simulink model "mavsim_chap3"  (R2021b)
settings: Solver=ode45  StartTime=0.0  StopTime=10000  RelTol=1e-3  EnableMultiTasking=on
InitFcn:
  | addpath('../chap2')
  | addpath('../parameters/')
  | aerosonde_parameters
undefined symbols (not defined in the file or in its folder): drawQuadrotor, plotmavstatevariables
libraries: simulink x7
settings Model: Creator=beard  LastModifiedBy=andrey
settings SolverCC: AlgebraicLoopSolver=TrustRegion
settings DataIOCC: LimitDataPoints=on  SaveFormat=Array  SignalLoggingSaveFormat=ModelDataLogs  ReturnWorkspaceOutputs=off
settings OptimizationCC: ExpressionDepthLimit=2147483647  InitFltsAndDblsToZero=on  LifeSpan=inf
settings DebuggingCC: UnderspecifiedInitializationDetection=Classic  MergeDetectMultiDrivingBlocksExec=none  SolverPrmCheckMsg=warning  FcnCallInpInsideContextMsg=warning  AllowSymbolicDim=off  StateNameClashWarn=warning  SFUnexpectedBacktrackingDiag=warning  SFNoUnconditionalDefaultTransitionDiag=warning  SFExecutionAtInitializationDiag=none  SFMachineParentedDataDiag=warning  ArithmeticOperatorsInVariantConditions=warning
settings HardwareCC: ProdBitPerPointer=32  ProdBitPerSizeT=32  ProdBitPerPtrDiffT=32  ProdLargestAtomicFloat=None  ProdIntDivRoundTo=Undefined  ProdEndianess=Unspecified  ProdWordSize=32  ProdHWDeviceType=32-bit Generic
settings ModelReferenceCC: PropagateSignalLabelsOutOfModel=off
settings SFSimCC: SimUseLocalCustomCode=off  CustomCodeUndefinedFunction=UseInterfaceOnly
settings RTWCC: RTWUseLocalCustomCode=off
settings CodeAppCC: StateflowObjectComments=on
settings GRTTargetCC: TargetLangStandard=C89/C90 (ANSI)  CombineOutputUpdateFcns=off  GRTInterface=on
settings ConfigComp: CovMetricSettings=dw  CovSaveCumulativeToWorkspaceVar=on  CovSaveSingleToWorkspaceVar=on  CovExternalEMLEnable=off  CovSFcnEnable=off

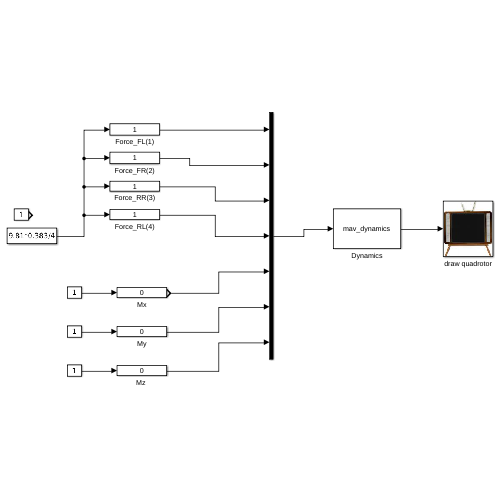
[thumbnail: Simulink's stored preview of the top-level diagram]
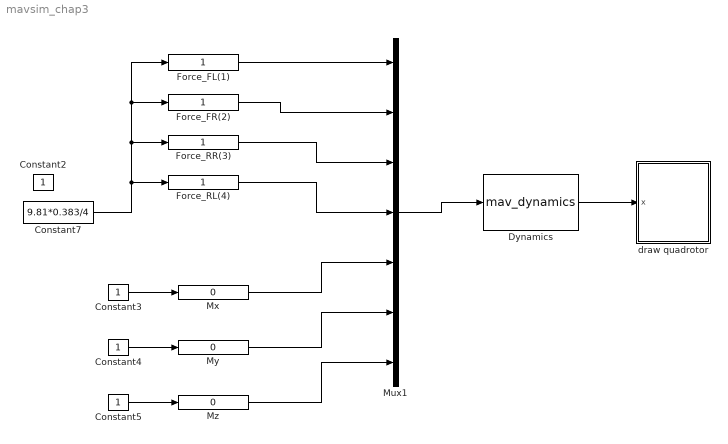
== system mavsim_chap3 ==
  Constant{2..5} (4 alike) : Constant
  Constant7 : Constant  Value=9.81*0.383/4
  Dynamics : S-Function  FunctionName=mav_dynamics  Parameters=MAV  SFunctionDeploymentMode=off  EnableBusSupport=off
  Force_FL(1) : simulink/Math Operations/Slider Gain  gain=1  low=0.999  high=1.001
  Force_FR(2) : simulink/Math Operations/Slider Gain  gain=1  low=0.999  high=1.001
  Force_RL(4) : simulink/Math Operations/Slider Gain  gain=1  low=0.999  high=1.001
  Force_RR(3) : simulink/Math Operations/Slider Gain  gain=1  low=0.999  high=1.001
  Mux1 : Mux  Inputs=7
  Mx : simulink/Math Operations/Slider Gain  gain=0  low=-1e-4  high=1e-4
  My : simulink/Math Operations/Slider Gain  gain=0  low=-1e-5  high=1e-5
  "Mz " : simulink/Math Operations/Slider Gain  gain=0  low=-1e-4  high=1e-4
  draw quadrotor : Subsystem
      mask Display: image(imread('../chap2/tv.jpg'))
  wires:
  Constant5/1 -> "Mz "/1
  Dynamics/1 -> draw quadrotor/1(x)
  Force_RL(4)/1 -> Mux1/4
  Force_RR(3)/1 -> Mux1/3
  Force_FL(1)/1 -> Mux1/1
  "Mz "/1 -> Mux1/7
  Constant4/1 -> My/1
  My/1 -> Mux1/6
  Constant3/1 -> Mx/1
  Mx/1 -> Mux1/5
  Mux1/1 -> Dynamics/1
  Force_FR(2)/1 -> Mux1/2
  Constant7/1 -> Force_RL(4)/1, Force_RR(3)/1, Force_FR(2)/1, Force_FL(1)/1

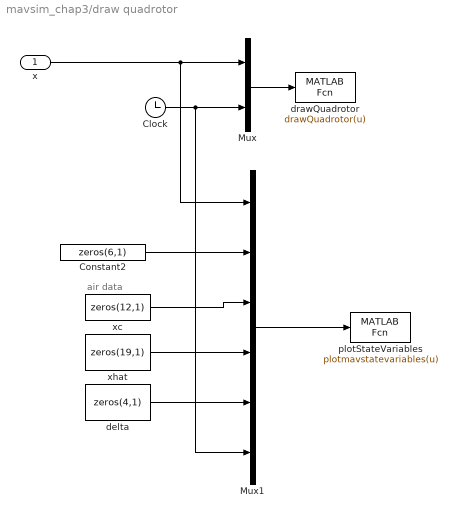
== system mavsim_chap3/draw quadrotor ==
  note: air data
  x : Inport
  Clock : Clock
  Constant2 : Constant  Value=zeros(6,1)
  Mux : Mux  Inputs=2
  Mux1 : Mux  Inputs=6
  delta : Constant  Value=zeros(4,1)
  drawQuadrotor : MATLABFcn  MATLABFcn=drawQuadrotor(u)  OutputDimensions=0  SampleTime=0.1
  plotStateVariables : MATLABFcn  MATLABFcn=plotmavstatevariables(u)  OutputDimensions=0
  xc : Constant  Value=zeros(12,1)
  xhat : Constant  Value=zeros(19,1)
  wires:
  x/1 -> Mux/1, Mux1/1
  Clock/1 -> Mux/2, Mux1/6
  Mux1/1 -> plotStateVariables/1
  xhat/1 -> Mux1/4
  xc/1 -> Mux1/3
  delta/1 -> Mux1/5
  Constant2/1 -> Mux1/2
  Mux/1 -> drawQuadrotor/1
